simulink model "ControlYPlanta"  (R2015a)
settings: Solver=ode45  StartTime=0.0  StopTime=inf  RelTol=1e-3
undefined symbols (not defined in the file or in its folder): serial
libraries: instrumentlib x3
settings Model: Creator=eduar  LastModifiedBy=eduar

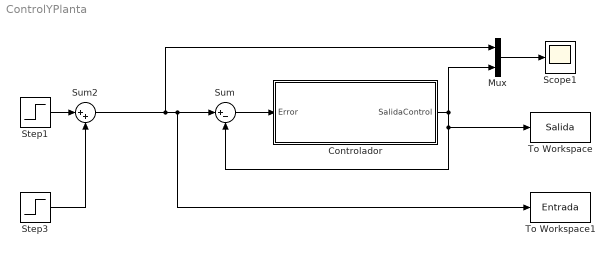
== system ControlYPlanta ==
  Controlador : Subsystem
  Mux : Mux  Inputs=2
  Scope1 : Scope
      settings: TimeRange=1000  YMin=10  YMax=95
  Step1 : Step  After=30  SampleTime=0
  Step3 : Step  Time=2000  After=40  SampleTime=0
  Sum : Sum  Inputs=|+-
  Sum2 : Sum  Inputs=|++
  To Workspace : ToWorkspace  VariableName=Salida  SampleTime=-1
      settings: Save2DSignal=2-D array (concatenate along first dimension)
  To Workspace1 : ToWorkspace  VariableName=Entrada  SampleTime=-1
      settings: Save2DSignal=2-D array (concatenate along first dimension)
  wires:
  Sum/1 -> Controlador/1(Error)
  Step1/1 -> Sum2/1
  Step3/1 -> Sum2/2
  Sum2/1 -> Mux/1, To Workspace1/1, Sum/1
  Mux/1 -> Scope1/1
  Controlador/1(SalidaControl) -> Sum/2, To Workspace/1, Mux/2

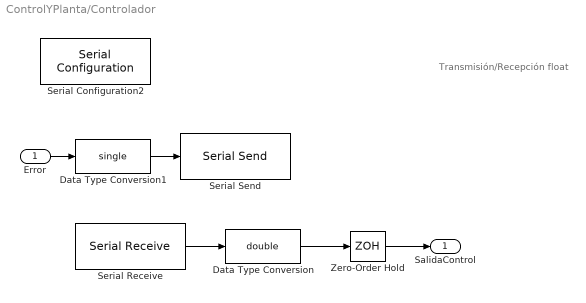
== system ControlYPlanta/Controlador ==
  note: Transmisión/Recepción float
  Error : Inport
  Data Type Conversion : DataTypeConversion  OutDataTypeStr=double  SampleTime=2
  Data Type Conversion1 : DataTypeConversion  OutDataTypeStr=single  SampleTime=2
  Serial Configuration2 : instrumentlib/Serial Configuration  Priority=-200000  ComPortMenu=COM5  ComPort=COM5  ObjConstructor=serial('COM5');  BaudRate=115200  DataBits=8  Parity=none  StopBits=1  FlowControl=none  Timeout=10  ByteOrder=LittleEndian
  Serial Receive : instrumentlib/Serial Receive  ComPortMenu=COM5  ComPort=COM5  ObjConstructor=serial('COM5');  Terminator=<none>  DataSize=[1 1]  DataType=single  EnableBlockingMode=on  ActionDataUnavailable=Output last received value  CustomValue=0  SampleTime=2
  Serial Send : instrumentlib/Serial Send  ComPortMenu=COM5  ComPort=COM5  ObjConstructor=serial('COM5');  Terminator=<none>  EnableBlockingMode=on
  Zero-Order Hold : ZeroOrderHold  SampleTime=2
  SalidaControl : Outport
  wires:
  Data Type Conversion/1 -> Zero-Order Hold/1
  Error/1 -> Data Type Conversion1/1
  Zero-Order Hold/1 -> SalidaControl/1
  Serial Receive/1 -> Data Type Conversion/1
  Data Type Conversion1/1 -> Serial Send/1
